simulink model "doc_oqpsk_modulation_delay"  (R2014a)
settings: Solver=FixedStepDiscrete  SolverMode=SingleTasking  StartTime=0.0  StopTime=1e3  RelTol=1e-3
undefined symbols (not defined in the file or in its folder): commblksprivate, Info
libraries: commdigbbndpm3 x2, commchan3 x1, commsink2 x1, commrandsrc2 x1
settings Model: Creator=The MathWorks Inc.
settings DataIOCC: SignalLoggingSaveFormat=ModelDataLogs
settings OptimizationCC: BlockReduction=off  BooleanDataType=off  ExpressionDepthLimit=2147483647  InitFltsAndDblsToZero=on
settings DebuggingCC: SaveWithParameterizedLinksMsg=none  UnderspecifiedInitializationDetection=Classic  SignalResolutionControl=TryResolveAllWithWarning  SolverPrmCheckMsg=none  MultiTaskDSMMsg=warning  MultiTaskCondExecSysMsg=none  FcnCallInpInsideContextMsg=UseLocalSettings  StateNameClashWarn=warning  StrictBusMsg=None
settings HardwareCC: TargetUnknown=on
settings RTWCC: IncludeERTFirstTime=on
settings GRTTargetCC: TargetFcnLib=ansi_tfl_tmw.mat  CombineOutputUpdateFcns=off  GRTInterface=on

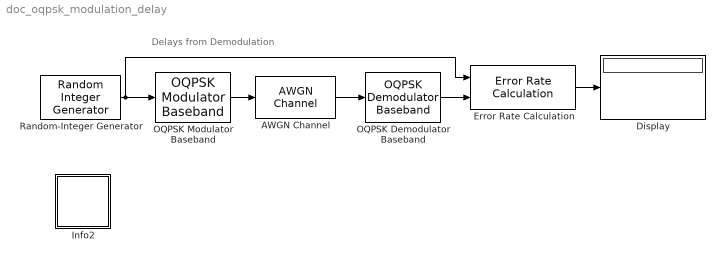
== system doc_oqpsk_modulation_delay ==
  note: Delays from Demodulation
  AWGN Channel : commchan3/AWGN Channel  InputProcessing=Columns as channels (frame based)  seed=67  noiseMode="Signal to noise ratio  (Es/No)"  EbNodB=10  EsNodB=6  SNRdB=10  bitsPerSym=1  Ps=1  Tsym=1  variance=1
  Display : Display
  Error Rate Calculation : commsink2/Error Rate Calculation  N=1  st_delay=0  cp_mode=Entire frame  subframe=[]  PMode=Port  WsName=ErrorVec  RsMode2=off  stop=off  numErr=100  maxBits=1e6
  Info2 : Subsystem  AncestorBlock=commblksprivate/Info  mask(Info){}
      settings: OpenFcn=helpview([docroot '/toolbox/comm/comm.map'], 'doc_oqpsk_modulation_delay')
      mask Display: disp('Info')
  OQPSK Demodulator Baseband : commdigbbndpm3/OQPSK Demodulator Baseband  OutType=Integer  Ph=0  RateOptions=Allow multirate processing  outDtype1=Inherit via internal rule  outDtype2=double  derotateFactorWordLen=16  roundingMode=Floor  overflowMode=Wrap
  OQPSK Modulator Baseband : commdigbbndpm3/OQPSK Modulator Baseband  InType=Integer  Ph=0  RateOptions=Allow multirate processing  outDtype=double  outWordLen=16  outUDDataType=sfix(16)  outFracLenMode=Best precision  outFracLen=15
  Random-Integer Generator : commrandsrc2/Random Integer Generator  mul=4  seed=10711  Ts=1  frameBased=off  sampPerFrame=1  orient=off  outDataType=double
  wires:
  Random-Integer Generator/1 -> Error Rate Calculation/1, OQPSK Modulator Baseband/1
  OQPSK Modulator Baseband/1 -> AWGN Channel/1
  OQPSK Demodulator Baseband/1 -> Error Rate Calculation/2
  Error Rate Calculation/1 -> Display/1
  AWGN Channel/1 -> OQPSK Demodulator Baseband/1

== system doc_oqpsk_modulation_delay/Info2 ==
